simulink model "SachinSharmaExample"  (R2020b)
settings: Solver=VariableStepAuto  StartTime=0.0  StopTime=10.0  RelTol=1e-3
settings Model: Creator=amazi  LastModifiedBy=amazi

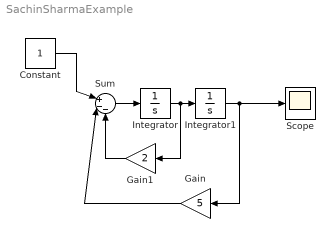
== system SachinSharmaExample ==
  Constant : Constant
  Gain : Gain  Gain=5
  Gain1 : Gain  Gain=2
  Integrator : Integrator
  Integrator1 : Integrator
  Scope : Scope
  Sum : Sum  Inputs=|+--
  wires:
  Constant/1 -> Sum/1
  Integrator1/1 -> Gain/1, Scope/1
  Gain/1 -> Sum/2
  Integrator/1 -> Integrator1/1, Gain1/1
  Sum/1 -> Integrator/1
  Gain1/1 -> Sum/3
